simulink model "NonLinearPatient_task5"  (R2022a)
settings: Solver=ode4  StartTime=0.0  StopTime=info.Tsim  FixedStep=0.1  RelTol=1e-15
values from neighbouring files (symbols this model uses):
  PH = 200    [MAIN_MIMO.m]    (also in backupMain.m; nonLinearPatient_main.m; test.m)
  R_KF = 0.001*eye(2)    [MAIN_MIMO.m]    (also in backupMain.m; nonLinearPatient_main.m; test.m)
  u_eq = [propofol_eq; remifentanil_eq]    [MAIN_MIMO.m]    (also in backupMain.m; nonLinearPatient_main.m; test.m)
  wantNoisyBIS = 1    [MAIN_MIMO.m]    (also in backupMain.m; nonLinearPatient_main.m; test.m)
  x_eq = operatingPoint.getstatestruct.signals.values    [MAIN_MIMO.m]    (also in backupMain.m; nonLinearPatient_main.m; test.m)
undefined symbols (not defined in the file or in its folder): DiscIntNeverNeededParam, discMat, Discrete, info, myMPC_dist, op, patient, propofol, RASS, remifentanil, Time
libraries: cstblocks x2, ctrlSharedLib x1
settings Model: Creator=cionescu  LastModifiedBy=user
settings SolverCC: AlgebraicLoopSolver=TrustRegion
settings DataIOCC: SaveState=on  ReturnWorkspaceOutputs=off
settings DebuggingCC: UnconnectedInputMsg=warning  UnconnectedOutputMsg=warning  UnconnectedLineMsg=warning  SFMachineParentedDataDiag=warning  ArithmeticOperatorsInVariantConditions=warning
settings SFSimCC: SimUseLocalCustomCode=off  CustomCodeUndefinedFunction=UseInterfaceOnly
settings RTWCC: RTWUseLocalCustomCode=off  DLArmComputeVersion=19.05
settings CodeAppCC: StateflowObjectComments=on

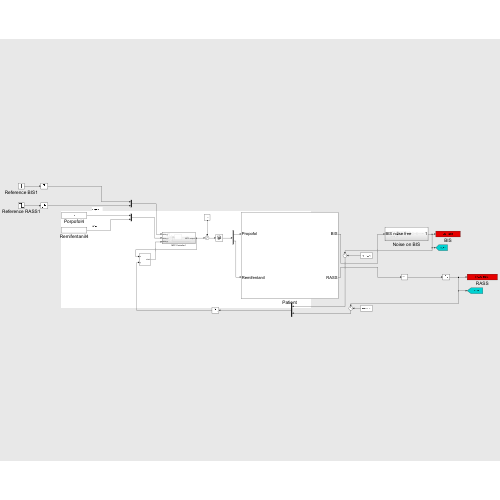
[thumbnail: Simulink's stored preview of the top-level diagram]
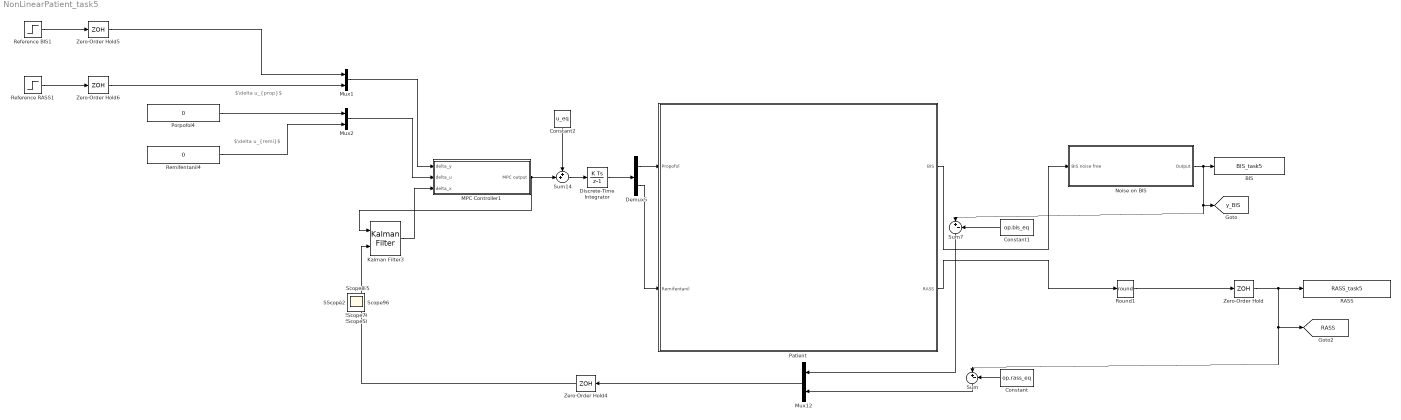
== system NonLinearPatient_task5 ==
  note: $\delta u_{remi}$
  note: $\delta u_{prop}$
  BIS : ToWorkspace  VariableName=BIS_task5  SaveFormat=Structure With Time  SampleTime=1
      settings: Save2DSignal=2-D array (concatenate along first dimension)
  Constant : Constant  Value=op.rass_eq
  Constant1 : Constant  Value=op.bis_eq
  Constant2 : Constant  Value=u_eq
  Demux5 : Demux  Outputs=2
  Discrete-Time Integrator : DiscreteIntegrator  SampleTime=info.Ts  ICPrevOutput=DiscIntNeverNeededParam  ICPrevScaledInput=DiscIntNeverNeededParam
  Kalman Filter3 : ctrlSharedLib/Kalman Filter  TimeDomain=Discrete-Time  UseCurrentEstimator=on  ModelSource=LTI State-Space Variable  ModelSourceVariable=discreteModel  A=0.95  B=1  C=1  D=0  NumberOfStates=1  NumberOfInputs=1  NumberOfOutputs=1  InitialEstimateSource=Dialog  X0=x_eq  P0=10  UseK=off  UseGH=off  NumberOfProcessNoiseInputs=1  G=1  TimeInvariantG=on  H=0  TimeInvariantH=on  Q=Q_KF  TimeInvariantQ=on  R=R_KF  TimeInvariantR=on  N=0  TimeInvariantN=on  AddInputPort=on  AddEnablePort=off  OutputEstimatedY=off  OutputP=off  Ts=-1
  MPC Controller1 : Subsystem
  Mux1 : Mux  Inputs=2
  Mux12 : Mux  Inputs=2
  Mux2 : Mux  Inputs=2
  Noise on BIS : Subsystem
  Patient : Subsystem
  Porpofol4 : Constant  Value=0  SampleTime=info.Ts
  RASS : ToWorkspace  VariableName=RASS_task5  SaveFormat=Structure With Time  SampleTime=1
      settings: Save2DSignal=2-D array (concatenate along first dimension)
  Reference BIS1 : Step  Time=info.T_induction  Before=50  After=0  SampleTime=info.Ts
  Reference RASS1 : Step  Time=info.T_induction  Before=4  After=0  SampleTime=info.Ts
  Remifentanil4 : Constant  Value=0  SampleTime=info.Ts
  Round1 : Rounding  Operator=round
  Sum : Sum  Inputs=|+-
  Sum14 : Sum  Inputs=++|
  Sum7 : Sum  Inputs=|+-
  Zero-Order Hold{,4..6} (4 alike) : ZeroOrderHold  SampleTime=info.Ts
  Scope{,2,5,7..16} (13 alike) : Scope
  tag scope: RASS=global, y_BIS=global
  wires:
  Sum14/1 -> Discrete-Time Integrator/1
  Zero-Order Hold4/1 -> Kalman Filter3/2
  Demux5/1 -> Patient/1(Propofol)
  Constant2/1 -> Sum14/1
  Demux5/2 -> Patient/2(Remifentanil)
  Round1/1 -> Zero-Order Hold/1
  Patient/2(RASS) -> Round1/1
  Patient/1(BIS) -> Noise on BIS/1(BIS noise free)
  Noise on BIS/1(Output) -> Sum7/1, [y_BIS], BIS/1
  Zero-Order Hold/1 -> Sum/1, [RASS], RASS/1
  Constant1/1 -> Sum7/2
  Sum7/1 -> Mux12/1
  Constant/1 -> Sum/2
  Sum/1 -> Mux12/2
  Mux12/1 -> Zero-Order Hold4/1
  Kalman Filter3/1 -> MPC Controller1/3(delta_x)
  Porpofol4/1 -> Mux2/1
  Reference RASS1/1 -> Zero-Order Hold6/1
  Zero-Order Hold5/1 -> Mux1/1
  Zero-Order Hold6/1 -> Mux1/2
  Mux2/1 -> MPC Controller1/2(delta_u)
  Mux1/1 -> MPC Controller1/1(delta_y)
  Remifentanil4/1 -> Mux2/2
  Reference BIS1/1 -> Zero-Order Hold5/1
  MPC Controller1/1(MPC output) -> Kalman Filter3/1, Sum14/2
  Discrete-Time Integrator/1 -> Demux5/1

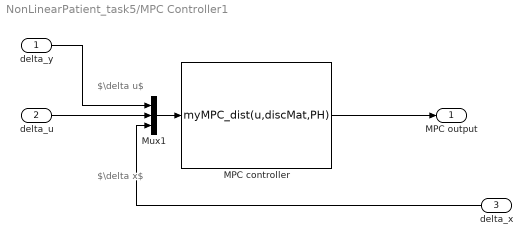
== system NonLinearPatient_task5/MPC Controller1 ==
  note: $\delta x$
  note: $\delta u$
  delta_y : Inport
  delta_u : Inport  Port=2
  delta_x : Inport  Port=3
  MPC controller : MATLABFcn  MATLABFcn=myMPC_dist(u,discMat,PH)  OutputDimensions=2
  Mux1 : Mux  Inputs=3
  MPC output : Outport
  wires:
  delta_x/1 -> Mux1/3
  Mux1/1 -> MPC controller/1
  MPC controller/1 -> MPC output/1
  delta_u/1 -> Mux1/2
  delta_y/1 -> Mux1/1

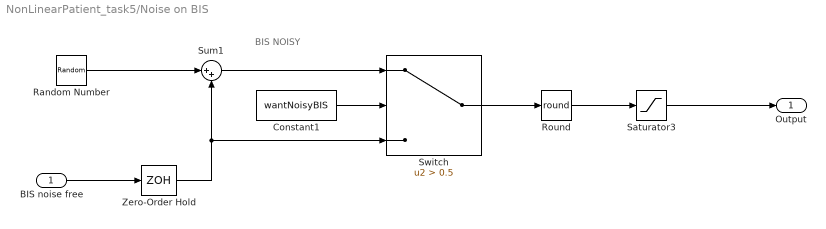
== system NonLinearPatient_task5/Noise on BIS ==
  note: BIS NOISY
  BIS noise free : Inport
  Constant1 : Constant  Value=wantNoisyBIS
  Random Number : RandomNumber  Variance=6.27  SampleTime=info.Ts
  Round : Rounding  Operator=round
  Saturator3 : Saturate  UpperLimit=100  LowerLimit=0
  Sum1 : Sum  Inputs=|++
  Switch : Switch  Criteria=u2 > Threshold  Threshold=0.5  SaturateOnIntegerOverflow=off  InputSameDT=off
  Zero-Order Hold : ZeroOrderHold  SampleTime=info.Ts
  Output : Outport
  wires:
  Round/1 -> Saturator3/1
  Random Number/1 -> Sum1/1
  Constant1/1 -> Switch/2
  Saturator3/1 -> Output/1
  Switch/1 -> Round/1
  BIS noise free/1 -> Zero-Order Hold/1
  Sum1/1 -> Switch/1
  Zero-Order Hold/1 -> Sum1/2, Switch/3

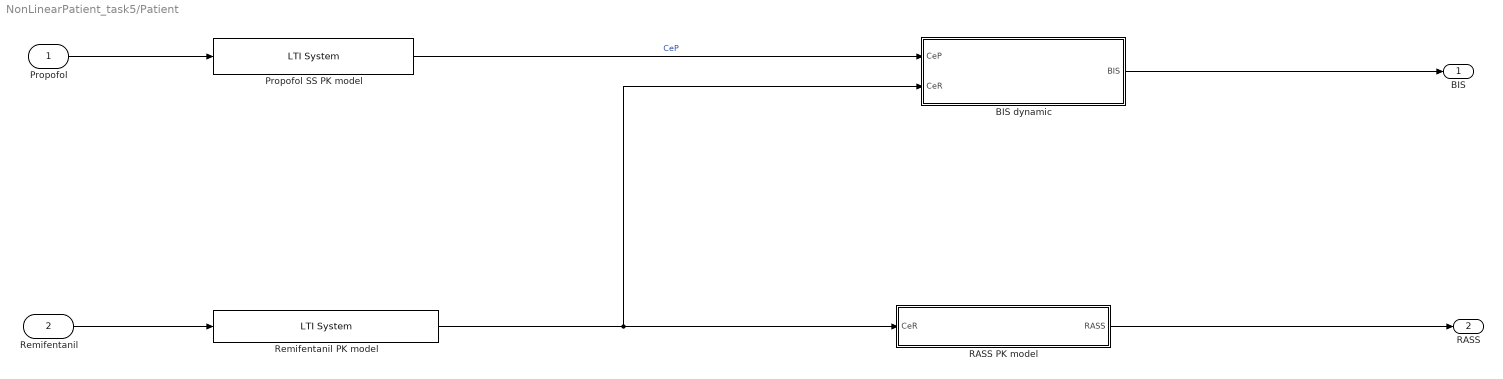
== system NonLinearPatient_task5/Patient ==
  Propofol : Inport
  Remifentanil : Inport  Port=2
  BIS dynamic : Subsystem
  Propofol SS PK model : cstblocks/LTI System  sys=propofol.propSS  IC=0
  RASS PK model : Subsystem
  Remifentanil PK model : cstblocks/LTI System  sys=remifentanil.remiSS  IC=0
  BIS : Outport
  RASS : Outport  Port=2
  wires:
  Propofol SS PK model/1 -> BIS dynamic/1(CeP)  "CeP"
  BIS dynamic/1(BIS) -> BIS/1
  Propofol/1 -> Propofol SS PK model/1
  Remifentanil/1 -> Remifentanil PK model/1
  Remifentanil PK model/1 -> RASS PK model/1(CeR), BIS dynamic/2(CeR)
  RASS PK model/1(RASS) -> RASS/1

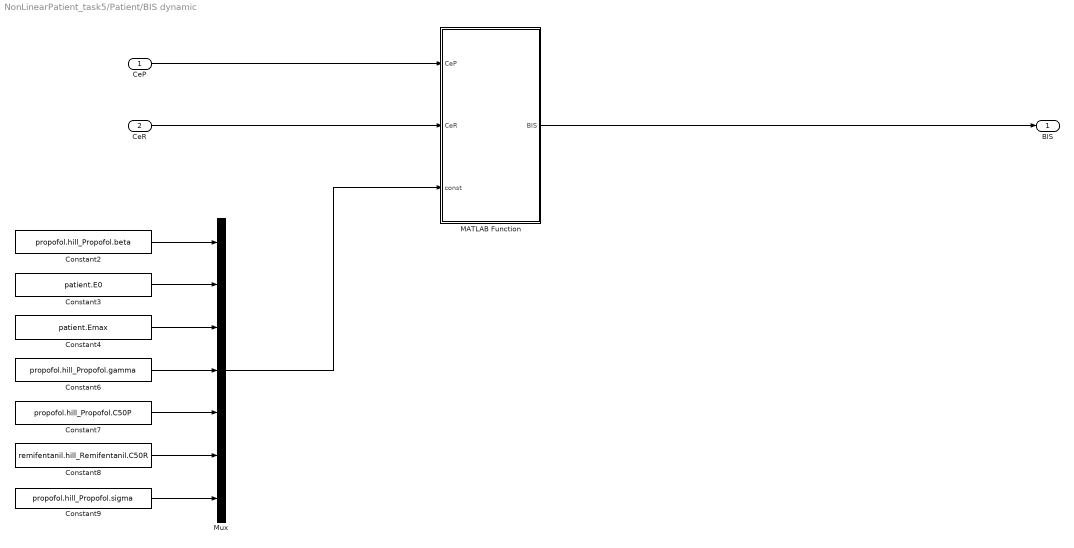
== system NonLinearPatient_task5/Patient/BIS dynamic ==
  CeP : Inport
  CeR : Inport  Port=2
  Constant2 : Constant  Value=propofol.hill_Propofol.beta
  Constant3 : Constant  Value=patient.E0
  Constant4 : Constant  Value=patient.Emax
  Constant6 : Constant  Value=propofol.hill_Propofol.gamma
  Constant7 : Constant  Value=propofol.hill_Propofol.C50P
  Constant8 : Constant  Value=remifentanil.hill_Remifentanil.C50R
  Constant9 : Constant  Value=propofol.hill_Propofol.sigma
  MATLAB Function : MATLAB Function  TreatAsAtomicUnit=on
  Mux : Mux  Inputs=7
  BIS : Outport
  wires:
  Constant9/1 -> Mux/7
  Constant8/1 -> Mux/6
  Constant4/1 -> Mux/3
  Mux/1 -> MATLAB Function/3(const)
  Constant7/1 -> Mux/5
  Constant3/1 -> Mux/2
  Constant6/1 -> Mux/4
  Constant2/1 -> Mux/1
  MATLAB Function/1(BIS) -> BIS/1
  CeP/1 -> MATLAB Function/1(CeP)
  CeR/1 -> MATLAB Function/2(CeR)

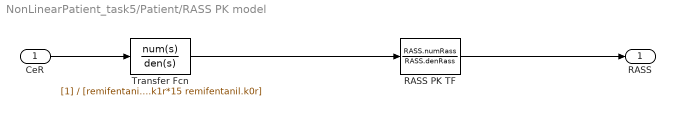
== system NonLinearPatient_task5/Patient/RASS PK model ==
  CeR : Inport
  RASS PK TF : TransferFcn  Numerator=RASS.numRass  Denominator=RASS.denRass
  Transfer Fcn : TransferFcn  Denominator=[remifentanil.k1r*15 remifentanil.k0r]
  RASS : Outport
  wires:
  CeR/1 -> Transfer Fcn/1
  Transfer Fcn/1 -> RASS PK TF/1
  RASS PK TF/1 -> RASS/1

== matlab function NonLinearPatient_task5/Patient/BIS dynamic/MATLAB Function ==
  data: CeP input; BIS output; CeR input; const input
function BIS = fcn(CeP,CeR, const)

if CeP >=0 && CeR >=0
    %% Constant declaration
    beta = const(1);
    E0 = const(2); %starting effect
%     E0 = const(2)-100; %starting effect
    Emax = const(3); %maximum effect achievable
    gamma = const(4); %sigmoidicity
    C50P = const(5); % half effect concentration
    C50R = const(6); % half effect concentration
    sigma = const(7);% sinergy between prop & rem
    
    %% 2D Calculations
    Uprop=CeP./C50P; Uremi=CeR./C50R;
    BIS=E0 - Emax*((Uprop)+(Uremi)+sigma*(Uprop)*(Uremi))^(gamma)/...
        (1+(Uprop+Uremi+sigma*Uprop*Uremi)^(gamma));

else
    BIS = 100;
end
